simulink model "New_saturationproperty"  (Simulink 7.9)
settings: Solver=FixedStepDiscrete  StartTime=0.0  StopTime=10  FixedStep=1  RelTol=1e-3
undefined symbols (not defined in the file): Carnot_saturationproperty_Callbacks
settings Model: Creator=awohlfei  LastModifiedBy=awohlfei

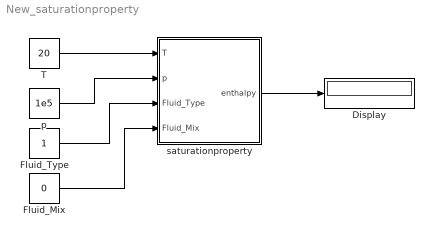
== system New_saturationproperty ==
  Display : Display
  Fluid_Mix : Constant  Value=0
  Fluid_Type : Constant
  T : Constant  Value=20
  p : Constant  Value=1e5
  saturationproperty : Subsystem  LoadFcn=Carnot_saturationproperty_Callbacks('LoadFcn');  InitFcn=load('THB.mat');  VariantObject=CarlibClassic  mask(saturation property){INPUTARGUMENTS=state variables (classic), PROPERTY=density, FLUIDPHASE=liquid, DEBUGLEVEL=WARNING, MAXTOTALMESSAGES=inf, MAXCONSECUTIVEMESSAGES=inf, WRITETOFILE=0, FILENAME='errors.txt'}
      mask prompts: INPUTARGUMENTS "Input arguments"; FLUIDPHASE "fluid phase"; DEBUGLEVEL "Debug level"; MAXTOTALMESSAGES "maximum number of total warning"; MAXCONSECUTIVEMESSAGES "maximum number of consecutive warnings"; WRITETOFILE "write messages to file"; FILENAME "filename for error messages"
      mask help:
      | The block calculates the saturation value of water by the value of a specified property. Calls the function "saturationproperty" in the CARNOT library "Carlib".
      |
      | PROPERTY            UNIT
      | density                     kg/m³
      | heat capacity           J/kgK
      | heat conductivity     W/mK
      | kinematic viscosity   m²/s
      | enthalpy                   J/kg
      | entropy                     J/kgK
      | prandtl                      --
      | specific volume        m³/kg
      mask init:
      | %Inports
      | Carnot_saturationproperty_Callbacks('CreateInports');
      | 
      | %global debug level
      | [DEBUGLEVEL, MAXTOTALMESSAGES, MAXCONSECUTIVEMESSAGES, WRITETOFILE, FILENAME] = Carnot_saturationproperty_Callbacks('CheckDebugLevels', DEBUGLEVEL, MAXTOTALMESSAGES, MAXCONSECUTIVEMESSAGES, WRITETOFILE, FILENAME);
      mask Help: eval('man(''saturationproperty'')')
      mask StyleString: popup(state variables (classic)|THB|THV),popup(density|heat capacity|heat conductivity|kinematic viscosity|enthalpy|entropy|prandtl|specific volume),popup(vaporous|liquid|solid),popup(DEBUG|INFO|WARNING|ERROR|FATAL|NONE),edit,edit,edit,edit
      mask CallbackString: Carnot_saturationproperty_Callbacks('MaskVisibilities');|||||||
      mask TabNameString: Parameters,Parameters,Parameters,Debugging,Debugging,Debugging,Debugging,Debugging
  wires:
  T/1 -> saturationproperty/1(T)
  p/1 -> saturationproperty/2(p)
  Fluid_Type/1 -> saturationproperty/3(Fluid_Type)
  Fluid_Mix/1 -> saturationproperty/4(Fluid_Mix)
  saturationproperty/1(enthalpy) -> Display/1

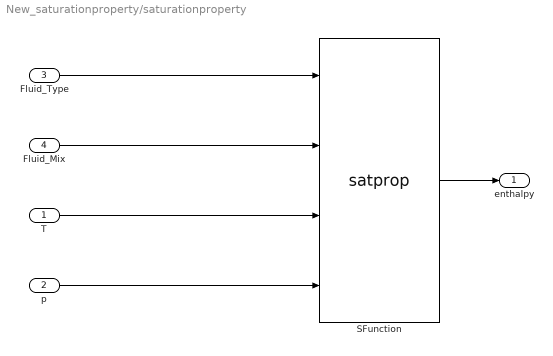
== system New_saturationproperty/saturationproperty ==
  T : Inport
  p : Inport  Port=2
  Fluid_Type : Inport  Port=3
  Fluid_Mix : Inport  Port=4
  SFunction : S-Function  FunctionName=satprop  Parameters=PROPERTY, FLUIDPHASE, DEBUGLEVEL, MAXTOTALMESSAGES, MAXCONSECUTIVEMESSAGES, WRITETOFILE, FILENAME  EnableBusSupport=off
  enthalpy : Outport
  wires:
  SFunction/1 -> enthalpy/1
  T/1 -> SFunction/3
  p/1 -> SFunction/4
  Fluid_Type/1 -> SFunction/1
  Fluid_Mix/1 -> SFunction/2
